simulink model "L4_rst_example_double_integrator"  (R2014b)
settings: Solver=ode45  StartTime=0.0  StopTime=10.0  RelTol=1e-3
values from neighbouring files (symbols this model uses):
  a_d = exp(a_c*h)    [L4_RST_spring16.m]
  h = findobj(gcf,'Type','line')    [AW_5_3.m]    (also in L4_RST_spring16.m = 0.1; PS4_ship_heading_RST_3h_script.m = 0.2; PS4_ship_heading_RST_noaa_script.m = 0.2; PS4_ship_heading_RST_script.m = 0.2)
  r1 = double(subs(sol.r1, vars, vals))    [AW_5_2.m]    (also in L4_RST_spring16.m = -0.856007930368168*a_d + 0.143992069631831; RST_example_spring18.m = params(1); hw5.m = -0.878368264722988*ea + 0.115597706410771)
  s0 = double(subs(sol.s0, vars, vals))    [AW_5_2.m]    (also in L4_RST_spring16.m = -28.7984139263664*a_d + 32.9380169529651; RST_example_spring18.m = params(2); hw5.m = -1.34327624390048*ea + 1.52396058689998)
  s1 = double(subs(sol.s1, vars, vals))    [AW_5_2.m]    (also in L4_RST_spring16.m = 24.6588108997672*a_d - 28.7984139263663; RST_example_spring18.m = params(3); hw5.m = 0.972399357505391*ea - 1.15308370050492)
  t0 = subs(Acs, z, 1) / subs(Bsa, z, 1)    [AW_5_3.m]    (also in L4_RST_spring16.m = 4.1396030266; RST_example_spring18.m = 0.210526315789; RST_sym.m = subs(Ac, z, 1) / subs(B, z, 1); RST_sym_handout.m = subs(Ac, z, 1) / subs(B, z, 1))
settings Model: Creator=kjartan  LastModifiedBy=kjartan

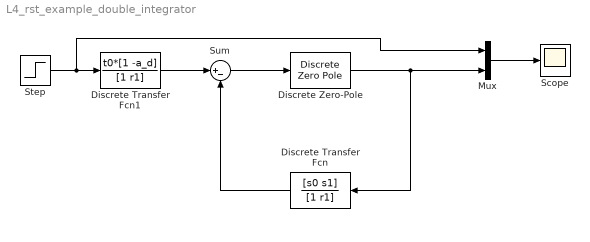
== system L4_rst_example_double_integrator ==
  Discrete Transfer Fcn : DiscreteTransferFcn  Numerator=[s0 s1]  Denominator=[1 r1]  SampleTime=h
  Discrete Transfer Fcn1 : DiscreteTransferFcn  Numerator=t0*[1 -a_d]  Denominator=[1 r1]  SampleTime=h
  Discrete Zero-Pole : DiscreteZeroPole  Zeros=[-1]  Poles=[1 1]  Gain=h^2/2  SampleTime=h
  Mux : Mux  Inputs=2
  Scope : Scope
  Step : Step  SampleTime=0
  Sum : Sum  Inputs=|+-
  wires:
  Discrete Zero-Pole/1 -> Discrete Transfer Fcn/1, Mux/2
  Sum/1 -> Discrete Zero-Pole/1
  Discrete Transfer Fcn1/1 -> Sum/1
  Discrete Transfer Fcn/1 -> Sum/2
  Step/1 -> Mux/1, Discrete Transfer Fcn1/1
  Mux/1 -> Scope/1
